simulink model "Schema_bloc"  (R2016a)
settings: Solver=VariableStepAuto  StartTime=0.0  StopTime=1000  RelTol=1e-3
values from neighbouring files (symbols this model uses):
  k = 0.035    [Prima_parte.m]
  k11 = k2^2+4*(k-k3)*k1    (= 0.0933546)    [Prima_parte.m]
  k12 = 8*(k-k3)    (= 0.2848)    [Prima_parte.m]
  k13 = 2*(k-k3)    (= 0.0712)    [Prima_parte.m]
  k2 = -0.015    [Prima_parte.m]
  keta = 8e-5    (= 8e-05)    [Prima_parte.m]
libraries: simulink x1
settings Model: Creator=Denisa  LastModifiedBy=catac

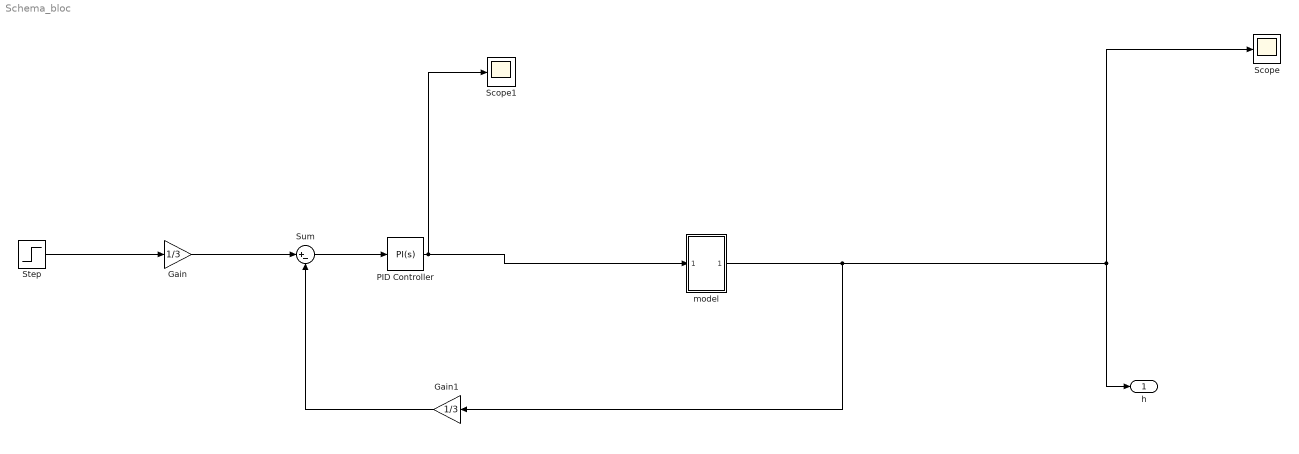
== system Schema_bloc ==
  Gain : Gain  Gain=1/3
  Gain1 : Gain  Gain=1/3
  PID Controller : simulink/Continuous/PID Controller  Controller=PI  TimeDomain=Continuous-time  SampleTime=-1  IntegratorMethod=Forward Euler  FilterMethod=Forward Euler  Form=Parallel  UseFilter=on  ControllerParametersSource=internal  P=2.395  I=0.0148  D=0  N=100  InitialConditionSource=internal  InitialConditionForIntegrator=5  InitialConditionForFilter=5  ExternalReset=none  LimitOutput=off  UpperSaturationLimit=inf  LowerSaturationLimit=-inf  LinearizeAsGain=on  AntiWindupMode=none  Kb=1  TrackingMode=off  Kt=1  PParamMin=[]  PParamMax=[]  IParamMin=[]  IParamMax=[]  DParamMin=[]  DParamMax=[]  NParamMin=[]  NParamMax=[]  KbParamMin=[]  KbParamMax=[]  KtParamMin=[]  KtParamMax=[]  POutMin=[]  POutMax=[]  IOutMin=[]  IOutMax=[]  DOutMin=[]  DOutMax=[]  NOutMin=[]  NOutMax=[]  KbOutMin=[]  KbOutMax=[]  KtOutMin=[]  KtOutMax=[]  IntegratorOutMin=[]  IntegratorOutMax=[]  FilterOutMin=[]  FilterOutMax=[]  SumOutMin=[]  SumOutMax=[]  SumI1OutMin=[]  SumI1OutMax=[]  SumI2OutMin=[]  SumI2OutMax=[]  SumI3OutMin=[]  SumI3OutMax=[]  SumDOutMin=[]  SumDOutMax=[]  SaturationOutMin=[]  SaturationOutMax=[]  IntegratorContinuousStateAttributes=''  IntegratorStateMustResolveToSignalObject=off  IntegratorRTWStateStorageClass=Auto  FilterContinuousStateAttributes=''  FilterStateMustResolveToSignalObject=off  FilterRTWStateStorageClass=Auto  DifferentiatorICPrevScaledInput=0  DifferentiatorOutMin=[]  DifferentiatorOutMax=[]
  Scope : Scope
  Scope1 : Scope
  Step : Step  Before=10  After=13.5  SampleTime=0
  Sum : Sum  Inputs=|+-
  model : Subsystem
  h : Outport
  wires:
  model/1(Out1) -> Gain1/1, h/1, Scope/1
  Step/1 -> Gain/1
  Gain/1 -> Sum/1
  Sum/1 -> PID Controller/1
  PID Controller/1 -> Scope1/1, model/1(In1)
  Gain1/1 -> Sum/2

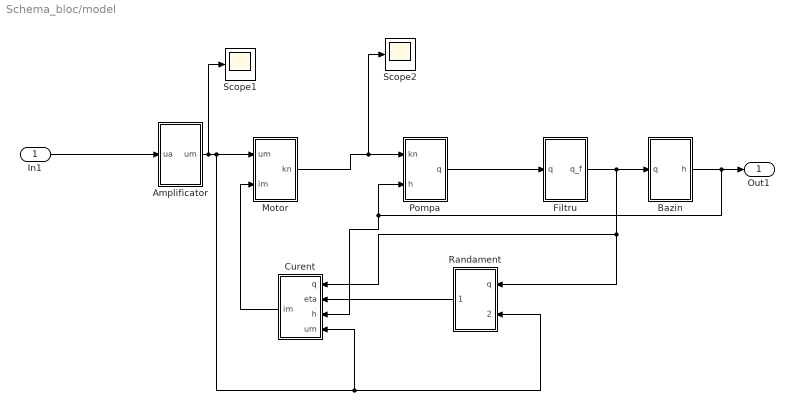
== system Schema_bloc/model ==
  In1 : Inport
  "Amplificator " : Subsystem
  "Bazin " : Subsystem
  "Curent " : Subsystem
  "Filtru " : Subsystem
  "Motor " : Subsystem
  "Pompa " : Subsystem
  "Randament " : Subsystem
  Scope1 : Scope
  Scope2 : Scope
  Out1 : Outport
  wires:
  "Filtru "/1("q_f ") -> "Curent "/1(q), "Randament "/1(q), "Bazin "/1("q ")
  "Bazin "/1("h ") -> Out1/1, "Curent "/3(h), "Pompa "/2(h)
  In1/1 -> "Amplificator "/1(ua)
  "Curent "/1(im) -> "Motor "/2(im)
  "Pompa "/1("q ") -> "Filtru "/1("q ")
  "Amplificator "/1(um) -> Scope1/1, "Curent "/4(um), "Randament "/2(um), "Motor "/1(um)
  "Motor "/1(kn) -> Scope2/1, "Pompa "/1(kn)
  "Randament "/1("eta ") -> "Curent "/2(eta)

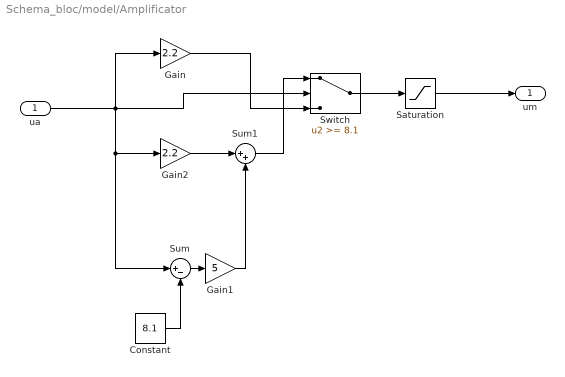
== system Schema_bloc/model/Amplificator  ==
  ua : Inport
  Constant : Constant  Value=8.1
  Gain : Gain  Gain=2.2
  Gain1 : Gain  Gain=5
  Gain2 : Gain  Gain=2.2
  Saturation : Saturate  UpperLimit=22  LowerLimit=0
  Sum : Sum  Inputs=|+-
  Sum1 : Sum  Inputs=|++
  Switch : Switch  Threshold=8.1  ZeroCross=off
  um : Outport
  wires:
  Gain1/1 -> Sum1/2
  Switch/1 -> Saturation/1
  Gain2/1 -> Sum1/1
  ua/1 -> Sum/1, Gain2/1, Gain/1, Switch/2
  Constant/1 -> Sum/2
  Sum/1 -> Gain1/1
  Saturation/1 -> um/1
  Gain/1 -> Switch/3
  Sum1/1 -> Switch/1

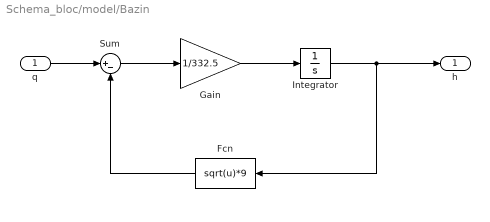
== system Schema_bloc/model/Bazin  ==
  "q " : Inport
  Fcn : Fcn  Expr=sqrt(u)*9
  Gain : Gain  Gain=1/332.5
  Integrator : Integrator  InitialCondition=10.5
  Sum : Sum  Inputs=|+-
  "h " : Outport
  wires:
  Gain/1 -> Integrator/1
  Fcn/1 -> Sum/2
  Sum/1 -> Gain/1
  "q "/1 -> Sum/1
  Integrator/1 -> "h "/1, Fcn/1

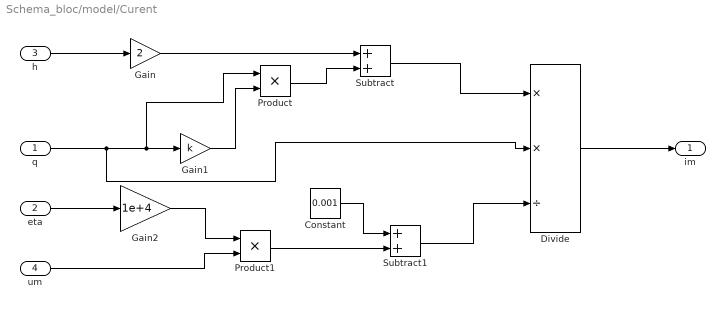
== system Schema_bloc/model/Curent  ==
  q : Inport
  eta : Inport  Port=2
  h : Inport  Port=3
  um : Inport  Port=4
  Constant : Constant  Value=0.001
  Divide : Product  Inputs=**/
  Gain : Gain  Gain=2
  Gain1 : Gain  Gain=k
  Gain2 : Gain  Gain=1e+4
  Product : Product
  Product1 : Product
  Subtract : Sum
  Subtract1 : Sum
  im : Outport
  wires:
  h/1 -> Gain/1
  q/1 -> Product/1, Gain1/1, Divide/2
  Product1/1 -> Subtract1/2
  Gain2/1 -> Product1/1
  Subtract/1 -> Divide/1
  um/1 -> Product1/2
  Constant/1 -> Subtract1/1
  Product/1 -> Subtract/2
  Subtract1/1 -> Divide/3
  eta/1 -> Gain2/1
  Gain/1 -> Subtract/1
  Gain1/1 -> Product/2
  Divide/1 -> im/1

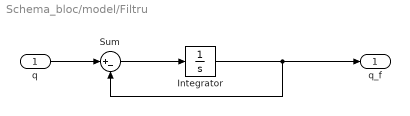
== system Schema_bloc/model/Filtru  ==
  "q " : Inport
  Integrator : Integrator  InitialCondition=29.2
  Sum : Sum  Inputs=|+-
  "q_f " : Outport
  wires:
  Integrator/1 -> "q_f "/1, Sum/2
  "q "/1 -> Sum/1
  Sum/1 -> Integrator/1

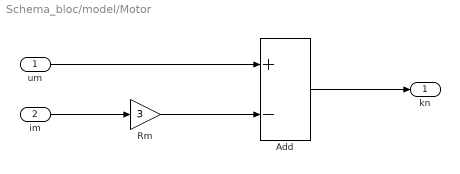
== system Schema_bloc/model/Motor  ==
  um : Inport
  im : Inport  Port=2
  Add : Sum  Inputs=+-
  Rm : Gain  Gain=3
  kn : Outport
  wires:
  Rm/1 -> Add/2
  im/1 -> Rm/1
  Add/1 -> kn/1
  um/1 -> Add/1

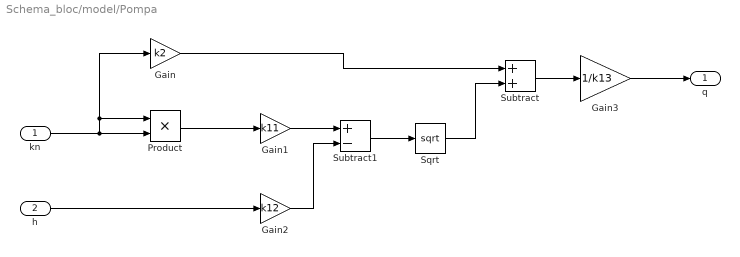
== system Schema_bloc/model/Pompa  ==
  kn : Inport
  h : Inport  Port=2
  Gain : Gain  Gain=k2
  Gain1 : Gain  Gain=k11
  Gain2 : Gain  Gain=k12
  Gain3 : Gain  Gain=1/k13
  Product : Product
  Sqrt : Sqrt  SaturateOnIntegerOverflow=on
  Subtract : Sum
  Subtract1 : Sum  Inputs=+-
  "q " : Outport
  wires:
  h/1 -> Gain2/1
  Product/1 -> Gain1/1
  Subtract/1 -> Gain3/1
  Gain3/1 -> "q "/1
  kn/1 -> Product/1, Gain/1, Product/2
  Gain1/1 -> Subtract1/1
  Gain2/1 -> Subtract1/2
  Gain/1 -> Subtract/1
  Sqrt/1 -> Subtract/2
  Subtract1/1 -> Sqrt/1

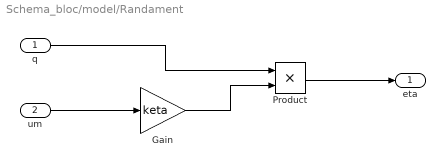
== system Schema_bloc/model/Randament  ==
  q : Inport
  um : Inport  Port=2
  Gain : Gain  Gain=keta
  Product : Product
  "eta " : Outport
  wires:
  q/1 -> Product/1
  Product/1 -> "eta "/1
  Gain/1 -> Product/2
  um/1 -> Gain/1
